simulink model "Bai2_R2016a"  (R2016a)
settings: Solver=ode5  SolverMode=SingleTasking  StartTime=0.0  StopTime=450  FixedStep=0.5  RelTol=1e-3
undefined symbols (not defined in the file): sigbuilder_block
libraries: fuzblock x1
settings Model: Creator=DELL  LastModifiedBy=DELL
settings DebuggingCC: SFUnexpectedBacktrackingDiag=error  SFNoUnconditionalDefaultTransitionDiag=error
settings GRTTargetCC: TargetLangStandard=C99 (ISO)  GeneratePreprocessorConditionals=Use local settings
settings ConfigComp: CovMetricSettings=dwe  CovHtmlReporting=off  CovSaveCumulativeToWorkspaceVar=off  CovSaveSingleToWorkspaceVar=off  CovExternalEMLEnable=on

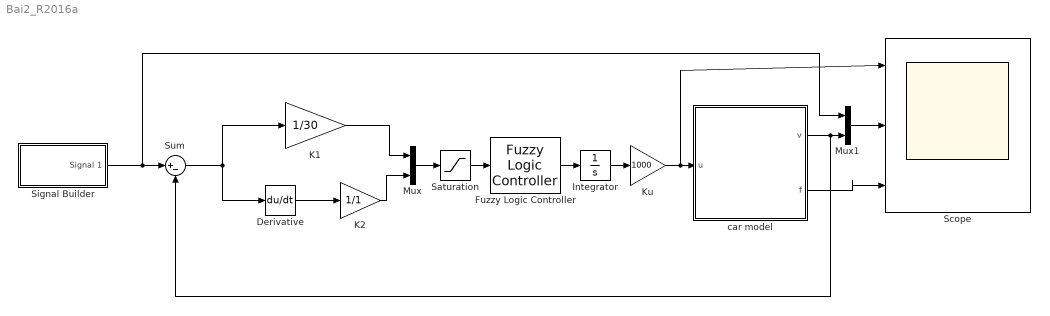
== system Bai2_R2016a ==
  Derivative : Derivative
  Fuzzy Logic Controller : fuzblock/Fuzzy Logic  Controller  FIS='fuzzy1.fis'
  Integrator : Integrator  LimitOutput=on  UpperSaturationLimit=1  LowerSaturationLimit=-1
  K1 : Gain  Gain=1/30
  K2 : Gain  Gain=1/1
  Ku : Gain  Gain=1000
  Mux : Mux  Inputs=2
  Mux1 : Mux  Inputs=2
  Saturation : Saturate  UpperLimit=1  LowerLimit=-1
  Scope : Scope  NumInputPorts=3
  Signal Builder : Subsystem  Tag=STV Subsys  LoadFcn=sigbuilder_block('load');  StartFcn=sigbuilder_block('start');  StopFcn=sigbuilder_block('stop');  ClipboardFcn=sigbuilder_block('clipboard');  mask(Sigbuilder block){}
      mask help: Simulink:masks:SigbuilderBlock_MD
      mask init:
      | if ~strcmp(get_param(bdroot(gcbh),'SimulationStatus'),'stopped') tuvar = sigbuilder_block('maskInit'); end
      settings: CopyFcn=sigbuilder_block('copy');  DeleteFcn=sigbuilder_block('delete');  ModelCloseFcn=sigbuilder_block('modelClose');  PreSaveFcn=sigbuilder_block('preSave');  PauseFcn=sigbuilder_block('pause');  ContinueFcn=sigbuilder_block('continue');  NameChangeFcn=sigbuilder_block('namechange');  OpenFcn=sigbuilder_block('open',[342.6 114.6 550.8 400.2 ]);  CloseFcn=sigbuilder_block('close');
      mask Display: plot(0, 0, 100, 100,[2, 2, 32, 32, 2], [68, 8, 8, 68, 68],[32, 2], [38, 38], [32, 19, 2],[53, 60, 44], [32, 17, 17, 2],[16, 16, 31, 31]);txt = getActiveGroup(gcbh);text(2, 100, txt,'verticalAlignment', 'top');
  Sum : Sum  Inputs=|+-
  car model : Subsystem  mask{A=0.3, m=1300, d=100, T=0.2}
  wires:
  Fuzzy Logic Controller/1 -> Integrator/1
  Mux/1 -> Saturation/1
  K1/1 -> Mux/1
  K2/1 -> Mux/2
  Sum/1 -> K1/1, Derivative/1
  Derivative/1 -> K2/1
  Ku/1 -> car model/1(u), Scope/1
  Integrator/1 -> Ku/1
  car model/1(v) -> Mux1/2, Sum/2
  Mux1/1 -> Scope/2
  Saturation/1 -> Fuzzy Logic Controller/1
  car model/2(f) -> Scope/3
  Signal Builder/1(Signal 1) -> Mux1/1, Sum/1

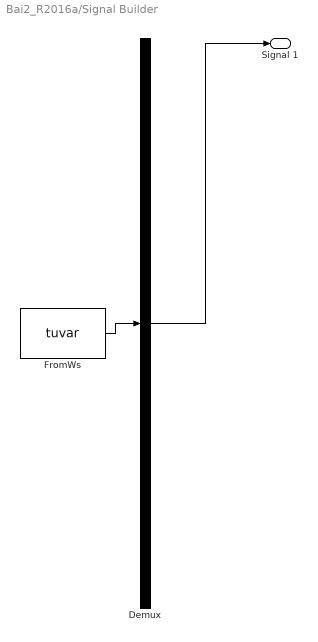
== system Bai2_R2016a/Signal Builder ==
  Demux : Demux  Tag=STV Demux  Outputs=1
  FromWs : FromWorkspace  Tag=STV FromWs  VariableName=tuvar  SampleTime=0
      SigBuilderData=|
      | common.afterFinalStr = 'Extrapolate'
      | common.sampleTime = 0
      | dataSet.timeRange = [0 450]
      | dataSet.name = 'Group 1'
      | sbobj.Groups.Name = 'Group 1'
      | sbobj.Groups.Signals.Name = 'Signal 1'
      | sbobj.Groups.Signals.XData = [0 75 75 151 151 226 226 300 300 376 376 450]
      | sbobj.Groups.Signals.YData = [30.2 30.2 20 20 9.8 9.8 25 25 15 15 30 30]
      | sbobj.Groups.TimeRange = [0 450]
  Signal 1 : Outport  Tag=STV Outport
  wires:
  Demux/1 -> Signal 1/1
  FromWs/1 -> Demux/1

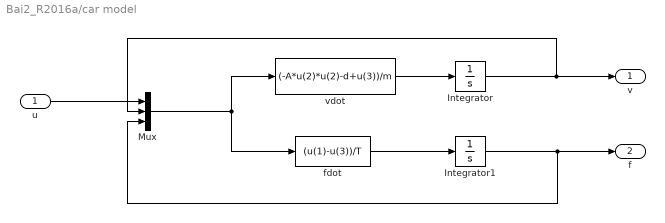
== system Bai2_R2016a/car model ==
  u : Inport
  "\tvdot " : Fcn  Expr=(-A*u(2)*u(2)-d+u(3))/m
  Integrator : Integrator
  Integrator1 : Integrator
  Mux : Mux  Inputs=3
  fdot : Fcn  Expr=(u(1)-u(3))/T
  v : Outport
  f : Outport  Port=2
  wires:
  "\tvdot "/1 -> Integrator/1
  Integrator/1 -> Mux/2, v/1
  u/1 -> Mux/1
  Mux/1 -> "\tvdot "/1, fdot/1
  fdot/1 -> Integrator1/1
  Integrator1/1 -> Mux/3, f/1
